simulink model "copy"  (R2024b)
settings: Solver=VariableStepAuto  StartTime=0.0  StopTime=5  RelTol=1e-3
settings Model: Creator=kiwiki  LastModifiedBy=kiwiki

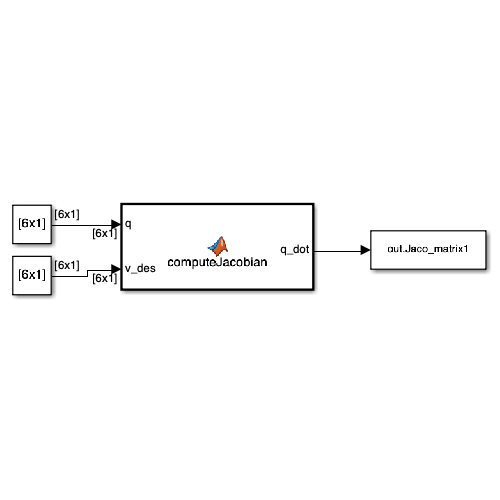
[thumbnail: Simulink's stored preview of the top-level diagram]
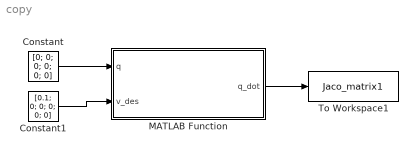
== system copy ==
  Constant : Constant  Value=[0; 0; 0; 0; 0; 0]  VectorParams1D=off  SampleTime=0.01
  Constant1 : Constant  Value=[0.1; 0; 0; 0; 0; 0]  VectorParams1D=off  SampleTime=0.01
  MATLAB Function : MATLAB Function  TreatAsAtomicUnit=on
  To Workspace1 : ToWorkspace  VariableName=Jaco_matrix1  SampleTime=0.01
      settings: Save2DSignal=2-D array (concatenate along first dimension)
  wires:
  MATLAB Function/1(q_dot) -> To Workspace1/1
  Constant/1 -> MATLAB Function/1(q)
  Constant1/1 -> MATLAB Function/2(v_des)

== matlab function copy/MATLAB Function ==
  data: q input; q_dot output; v_des input
function q_dot = computeJacobian(q, v_des)
coder.extrinsic('geometricJacobian');
coder.extrinsic('loadrobot');

% 預先定義輸出大小，避免 Simulink 無法推斷維度
q_dot = zeros(6,1); 

% 讀取機械手臂模型
robot = loadrobot('universalUR5', 'DataFormat', 'column');

% 計算雅可比矩陣
J = geometricJacobian(robot, q, 'tool0');

% 確保 J 不是空的
if ~isempty(J)
    % 計算雅可比偽逆
    J_pinv = pinv(J);

    % 計算關節速度 q_dot = J_pinv * v_des
    q_dot = J_pinv * v_des;
end
end
